simulink model "ACCSampleSimulink"  (R2022a)
settings: Solver=ode1  StartTime=0.0  StopTime=inf  FixedStep=0.001  RelTol=1e-3
model workspace (MAT data in the model file):
  ParaDataStoreNum : Simulink.Parameter (value not decoded)
undefined symbols (not defined in the file): azimuth_angle, DataStoreNumPara, elevation_angle, GroundTruth_Objects, heading, id, range_bbox, range_center, shape, time, type, velocity, width
(part 2 of 2)

== matlab function ACCSampleSimulink/Veh_1/ComplexVehicleModel/RoadInfo/MATLAB Function ==
  data: fl input; tire_x output; fr input; rl input; rr input; tire_y output; tire_z output
function [tire_x,tire_y,tire_z] = fcn(fl,fr,rl,rr)

tire_x = [fl(11),fr(11),rl(11),rr(11)];
tire_y = [fl(12),fr(12),rl(12),rr(12)];
tire_z = [fl(13),fr(13),rl(13),rr(13)];

== matlab function ACCSampleSimulink/Veh_1/ComplexVehicleModel/RoadInfo/MATLAB Function1 ==
  data: t input; outz output; z input; dzdx input; dzdy input; mu input; tirez input; outdzdx output; outdzdy output; outmu output
function [outz,outdzdx,outdzdy,outmu] = fcn(t,z,dzdx,dzdy,mu,tirez)
%#codegen
outz = tirez;
outdzdx = [0,0,0,0];
outdzdy = [0,0,0,0];
outmu = [0.75,0.75,0.75,0.75];
if t > 0.001
    outz = z;
    outdzdx = dzdx;
    outdzdy = dzdy;
    outmu = mu;
end

== matlab function ACCSampleSimulink/Veh_1/VehicleDataBus/MATLAB Function ==
  data: u input; head output; c_x output; c_y output; c_z output; yaw output; pitch output; roll output; rot_spd output; f_x output; f_y output; f_z output; g_x output; g_y output; g_z output
function [head,c_x,c_y,c_z,yaw,pitch,roll,rot_spd,f_x,f_y,f_z,g_x,g_y,g_z] = fcn(u)
head = [u(1),u(2),u(3),u(4),u(5)];
start = 6;
c_x =   [u(start),u(start+13),u(start+26),u(start+39)];
start = 7;
c_y =   [u(start),u(start+13),u(start+26),u(start+39)];
start = 8;
c_z =   [u(start),u(start+13),u(start+26),u(start+39)];
start = 9;
yaw =   [u(start),u(start+13),u(start+26),u(start+39)];
start = 10;
pitch = [u(start),u(start+13),u(start+26),u(start+39)];
start = 11;
roll =  [u(start),u(start+13),u(start+26),u(start+39)];
start = 12;
rot_spd =  [u(start),u(start+13),u(start+26),u(start+39)];
start = 13;
f_x =  [u(start),u(start+13),u(start+26),u(start+39)];
start = 14;
f_y =  [u(start),u(start+13),u(start+26),u(start+39)];
start = 15;
f_z =  [u(start),u(start+13),u(start+26),u(start+39)];
start = 16;
g_x =  [u(start),u(start+13),u(start+26),u(start+39)];
start = 17;
g_y =  [u(start),u(start+13),u(start+26),u(start+39)];
start = 18;
g_z =  [u(start),u(start+13),u(start+26),u(start+39)];

== matlab function ACCSampleSimulink/Veh_1/ComplexVehicleModel/MATLAB Function1 ==
  data: u input; ego output; egoextra output
function [ego,egoextra] = fcn(u)

ego = [u(2),u(3),u(4),u(5),u(6),u(7),u(8)];
egoextra = [u(8),u(9),u(10),u(11),u(12),u(13),u(14),u(15),u(16),u(17),u(18),u(19)];

== matlab function ACCSampleSimulink/Veh_1/ComplexVehicleModel/MATLAB Function2 ==
  data: driverControl input; throttle output; dynamicControl input; brake output; steer output; mode output
function [throttle,brake,steer,mode] = fcn(driverControl,dynamicControl)
%#codegen
if driverControl(1) > 0.5
    throttle = driverControl(2);
    brake = driverControl(3)* 1e6;
    steer = driverControl(4) * 0.0174;
    mode = driverControl(5);
else
    throttle = dynamicControl(3);
    brake = dynamicControl(4);
    steer = dynamicControl(5);
    mode = dynamicControl(2);
end

if mode > 0.5
   mode = 1 ;
end

== matlab function ACCSampleSimulink/Veh_1/Algorithm/ Find Leader Car/Find Leader Car ==
  data: EGOX input; RelatedDistance output; EGOY input; EGOV input; EGOYAW input; time input; width input; ids input; types input; shapes input; range_centers input; range_bboxs input; azimuth_angles input; elevation_angles input; velocitys input; headings input; RelatedSpeed output
function [RelatedDistance, RelatedSpeed]  = DetectionConcatenation(EGOX,EGOY,EGOV, EGOYAW, time, width, ids, types, shapes, range_centers, range_bboxs, azimuth_angles, elevation_angles, velocitys, headings)


% This function finds the lead car: a car in front of the ego car that
% satisfies all the criteria below:
% * Within the ego car's lane.
% * In front of the ego car.
% * Closest to the ego car.


% 1. The lane is defined using a parabolic model, where y=ax^2+bx+c. a is
%    equal to half the road curvature, b=0, and c is the offset of the lane
%    boundaries relative to the ego car. Overall lane width is assumed to
%    be 3.6m, typical highway lane width.
laneWidth = 3.6;

% 2. The ego car is assumed to be traveling in the middle of its lane, with
%    1.8m on each side of it. So, c=+1.8m for the left lane boundary and
%    -1.8m for the right lane boundary.
halfLaneWidth = laneWidth/2;

maxX = cast(500.0,'double');
Selected = cast(-1,'int32');

if(width > 0)
    for i = 1:width
        dis = range_bboxs(i);
        speed = velocitys(i);
        angle = -azimuth_angles(i);
        yaw = 3.1415926/2 - headings(i);
        deltaYaw = yaw - EGOYAW;
        x = dis * cos(angle); % Longitudinal position of the track relative to ego
        y = dis * sin(angle); % Lateral position of the track relative to ego
        if dis < maxX && dis > 0
            yleftLane  = polyval([0, 0,  halfLaneWidth],x); % Half a lane to the left
            yrightLane = polyval([0, 0, -halfLaneWidth],x); % Half a lane to the right

            % Find a new lead car
            if(yrightLane <= y) && (y<=yleftLane)
                maxX = cast(dis,'double');
                Selected = i;
            end
        end
    end
end

if(Selected ~= -1)
    RelatedDistance = cast(range_bboxs(Selected),'double');
    yaw = 3.1415926/2 - headings(Selected);
    speed = velocitys(Selected);
    deltaYaw = yaw - EGOYAW;
    Vxx = speed * cos(deltaYaw);
    %Vyy = speed * sin(deltaYaw);
    RelatedSpeed = cast(-EGOV + Vxx,'double');
else
    RelatedDistance = 500;
    RelatedSpeed = 0.1;
end

== matlab function ACCSampleSimulink/Veh_1/ComplexVehicleModel/RoadInfo/Subsystem/front_right ==
  data: out output double; xarry input; yarray input; zarray input; dzdxarray input; dzdyarray input; muarray input; x input; y input
function out  = fcn(xarry,yarray,zarray,dzdxarray,dzdyarray,muarray,x,y)
[x1,y1,x2,y2,x3,y3,x4,y4] = fcn_getpoint(xarry,yarray);
data_array = fcn_getdata(zarray,dzdxarray, dzdyarray,muarray);

zero = 0.001;
if ( abs(y2-y1) > zero )
   angle = 2*pi -  atan2(y2-y1,x2-x1);
   sin_angle = sin(angle);
   cos_angle = cos(angle);
   [x1,y1] = fcn_convert(x1,y1,x1,y1,sin_angle,cos_angle);
   [x2,y2] = fcn_convert(x1,y1,x2,y2,sin_angle,cos_angle);
   [x3,y3] = fcn_convert(x1,y1,x3,y3,sin_angle,cos_angle);
   [x4,y4] = fcn_convert(x1,y1,x4,y4,sin_angle,cos_angle);
   [x,y] = fcn_convert(x1,y1,x,y,sin_angle,cos_angle);
end

axle_x_left  = min(x1,x2);
axle_x_right = max(x1,x2);
axle_y_up    = max(y2,y3);
axle_y_down  = min(y2,y3);

% after rotota
% p1  p2
%
% p3 p4
z = 0;
dzdx = 0;
dzdy = 0;
mu = 0;
if ( x > axle_x_left ) && ( x < axle_x_right ) && ( y > axle_y_down ) && ( y < axle_y_up )
    xx1 = x3;
    xx2 = x4;
    yy1 = y3;
    yy2 = y1;
    matrix_left = [xx2-x  x-xx1];
    matrix_right = [ yy2 - y; y-yy1 ];
    delta = (xx2-xx1)*(yy2-yy1);
    delta = 1.0/delta;
    [z, dzdx, dzdy, mu] = fcn_cal(matrix_left,matrix_right,delta,data_array);
else
    if ( y >= axle_y_up ) 
        [z, dzdx, dzdy, mu] = fcn_cal_getmax(data_array(1,:),data_array(2,:));
    end
    if ( y <= axle_y_down )
        [z, dzdx, dzdy, mu] = fcn_cal_getmax(data_array(3,:),data_array(4,:));
    end
    if ( x >= axle_x_right )
        [z, dzdx, dzdy, mu] = fcn_cal_getmax(data_array(2,:),data_array(4,:));
    end
    if ( x <= axle_x_left )
        [z, dzdx, dzdy, mu] = fcn_cal_getmax(data_array(1,:),data_array(3,:));
    end
end

out = [z dzdx dzdy mu];
end

function [xxx,yyy] = fcn_convert(x0,y0,x1,y1,sin_agnle,cos_angle)
    xxx = (x1-x0)*cos_angle - (y1-y0)*sin_agnle + x0;
    yyy = (x1-x0)*sin_agnle + (y1-y0)*cos_angle + y0;
end

function [x1,y1,x2,y2,x3,y3,x4,y4] = fcn_getpoint(xarry,yarray)
    x1 = xarry(1);
    x2 = xarry(2);
    x3 = xarry(3);
    x4 = xarry(4);
    y1 = yarray(1);
    y2 = yarray(2);
    y3 = yarray(3);
    y4 = yarray(4);
end

function ret = fcn_getdata(zarray,dzdxarray, dzdyarray,muarray)
    ret = [ 
        zarray(1),dzdxarray(1),dzdyarray(1),muarray(1);
        zarray(2),dzdxarray(2),dzdyarray(2),muarray(2);
        zarray(3),dzdxarray(3),dzdyarray(3),muarray(3);
        zarray(4),dzdxarray(4),dzdyarray(4),muarray(4);
    ];
end

function [z,dzdx,dzdy,mu] = fcn_cal(matrix_left,matrix_right , delta, data_array)
%matrix_z = [z3, z1; z4 , z2]
%value = [xx2-x  x-xx1] * matrix * [ yy2 - y; y-yy1 ]  * d1
    array_z = data_array(:,1);
    array_dzdx = data_array(:,2);
    array_dzdy = data_array(:,3);
    array_mu = data_array(:,4);
    z = matrix_left * [array_z(3), array_z(1); array_z(4),array_z(2)] * matrix_right  * delta;
    dzdx = matrix_left * [array_dzdx(3), array_dzdx(1); array_dzdx(4),array_dzdx(2)] * matrix_right  * delta;
    dzdy = matrix_left * [array_dzdy(3), array_dzdy(1); array_dzdy(4),array_dzdy(2)] * matrix_right  * delta;
    mu = matrix_left * [array_mu(3), array_mu(1); array_mu(4),array_mu(2)] * matrix_right  * delta;
end

function [z,dzdx,dzdy,mu] = fcn_cal_getmax(data1,data2)
    z = max(data1(1),data2(1));
    dzdx = max(data1(2),data2(2));
    dzdy = max(data1(3),data2(3));
    mu = max(data1(4),data2(4));
end

== matlab function ACCSampleSimulink/Veh_1/ComplexVehicleModel/RoadInfo/Subsystem/front_left ==
  data: out output double; xarry input; yarray input; zarray input; dzdxarray input; dzdyarray input; muarray input; x input; y input
function out  = fcn(xarry,yarray,zarray,dzdxarray,dzdyarray,muarray,x,y)
[x1,y1,x2,y2,x3,y3,x4,y4] = fcn_getpoint(xarry,yarray);
data_array = fcn_getdata(zarray,dzdxarray, dzdyarray,muarray);

zero = 0.001;
if ( abs(y2-y1) > zero )
   angle = 2*pi -  atan2(y2-y1,x2-x1);
   sin_angle = sin(angle);
   cos_angle = cos(angle);
   [x1,y1] = fcn_convert(x1,y1,x1,y1,sin_angle,cos_angle);
   [x2,y2] = fcn_convert(x1,y1,x2,y2,sin_angle,cos_angle);
   [x3,y3] = fcn_convert(x1,y1,x3,y3,sin_angle,cos_angle);
   [x4,y4] = fcn_convert(x1,y1,x4,y4,sin_angle,cos_angle);
   [x,y] = fcn_convert(x1,y1,x,y,sin_angle,cos_angle);
end

axle_x_left  = min(x1,x2);
axle_x_right = max(x1,x2);
axle_y_up    = max(y2,y3);
axle_y_down  = min(y2,y3);

% after rotota
% p1  p2
%
% p3 p4
z = 0;
dzdx = 0;
dzdy = 0;
mu = 0;
if ( x > axle_x_left ) && ( x < axle_x_right ) && ( y > axle_y_down ) && ( y < axle_y_up )
    xx1 = x3;
    xx2 = x4;
    yy1 = y3;
    yy2 = y1;
    matrix_left = [xx2-x  x-xx1];
    matrix_right = [ yy2 - y; y-yy1 ];
    delta = (xx2-xx1)*(yy2-yy1);
    delta = 1.0/delta;
    [z, dzdx, dzdy, mu] = fcn_cal(matrix_left,matrix_right,delta,data_array);
else
    if ( y >= axle_y_up ) 
        [z, dzdx, dzdy, mu] = fcn_cal_getmax(data_array(1,:),data_array(2,:));
    end
    if ( y <= axle_y_down )
        [z, dzdx, dzdy, mu] = fcn_cal_getmax(data_array(3,:),data_array(4,:));
    end
    if ( x >= axle_x_right )
        [z, dzdx, dzdy, mu] = fcn_cal_getmax(data_array(2,:),data_array(4,:));
    end
    if ( x <= axle_x_left )
        [z, dzdx, dzdy, mu] = fcn_cal_getmax(data_array(1,:),data_array(3,:));
    end
end

out = [z dzdx dzdy mu];
end

function [xxx,yyy] = fcn_convert(x0,y0,x1,y1,sin_agnle,cos_angle)
    xxx = (x1-x0)*cos_angle - (y1-y0)*sin_agnle + x0;
    yyy = (x1-x0)*sin_agnle + (y1-y0)*cos_angle + y0;
end

function [x1,y1,x2,y2,x3,y3,x4,y4] = fcn_getpoint(xarry,yarray)
    x1 = xarry(1);
    x2 = xarry(2);
    x3 = xarry(3);
    x4 = xarry(4);
    y1 = yarray(1);
    y2 = yarray(2);
    y3 = yarray(3);
    y4 = yarray(4);
end

function ret = fcn_getdata(zarray,dzdxarray, dzdyarray,muarray)
    ret = [ 
        zarray(1),dzdxarray(1),dzdyarray(1),muarray(1);
        zarray(2),dzdxarray(2),dzdyarray(2),muarray(2);
        zarray(3),dzdxarray(3),dzdyarray(3),muarray(3);
        zarray(4),dzdxarray(4),dzdyarray(4),muarray(4);
    ];
end

function [z,dzdx,dzdy,mu] = fcn_cal(matrix_left,matrix_right , delta, data_array)
%matrix_z = [z3, z1; z4 , z2]
%value = [xx2-x  x-xx1] * matrix * [ yy2 - y; y-yy1 ]  * d1
    array_z = data_array(:,1);
    array_dzdx = data_array(:,2);
    array_dzdy = data_array(:,3);
    array_mu = data_array(:,4);
    z = matrix_left * [array_z(3), array_z(1); array_z(4),array_z(2)] * matrix_right  * delta;
    dzdx = matrix_left * [array_dzdx(3), array_dzdx(1); array_dzdx(4),array_dzdx(2)] * matrix_right  * delta;
    dzdy = matrix_left * [array_dzdy(3), array_dzdy(1); array_dzdy(4),array_dzdy(2)] * matrix_right  * delta;
    mu = matrix_left * [array_mu(3), array_mu(1); array_mu(4),array_mu(2)] * matrix_right  * delta;
end

function [z,dzdx,dzdy,mu] = fcn_cal_getmax(data1,data2)
    z = max(data1(1),data2(1));
    dzdx = max(data1(2),data2(2));
    dzdy = max(data1(3),data2(3));
    mu = max(data1(4),data2(4));
end

== matlab function ACCSampleSimulink/Veh_1/ComplexVehicleModel/RoadInfo/Subsystem/tail_left ==
  data: out output double; xarry input; yarray input; zarray input; dzdxarray input; dzdyarray input; muarray input; x input; y input
function out  = fcn(xarry,yarray,zarray,dzdxarray,dzdyarray,muarray,x,y)
[x1,y1,x2,y2,x3,y3,x4,y4] = fcn_getpoint(xarry,yarray);
data_array = fcn_getdata(zarray,dzdxarray, dzdyarray,muarray);

zero = 0.001;
if ( abs(y2-y1) > zero )
   angle = 2*pi -  atan2(y2-y1,x2-x1);
   sin_angle = sin(angle);
   cos_angle = cos(angle);
   [x1,y1] = fcn_convert(x1,y1,x1,y1,sin_angle,cos_angle);
   [x2,y2] = fcn_convert(x1,y1,x2,y2,sin_angle,cos_angle);
   [x3,y3] = fcn_convert(x1,y1,x3,y3,sin_angle,cos_angle);
   [x4,y4] = fcn_convert(x1,y1,x4,y4,sin_angle,cos_angle);
   [x,y] = fcn_convert(x1,y1,x,y,sin_angle,cos_angle);
end

axle_x_left  = min(x1,x2);
axle_x_right = max(x1,x2);
axle_y_up    = max(y2,y3);
axle_y_down  = min(y2,y3);

% after rotota
% p1  p2
%
% p3 p4
z = 0;
dzdx = 0;
dzdy = 0;
mu = 0;
if ( x > axle_x_left ) && ( x < axle_x_right ) && ( y > axle_y_down ) && ( y < axle_y_up )
    xx1 = x3;
    xx2 = x4;
    yy1 = y3;
    yy2 = y1;
    matrix_left = [xx2-x  x-xx1];
    matrix_right = [ yy2 - y; y-yy1 ];
    delta = (xx2-xx1)*(yy2-yy1);
    delta = 1.0/delta;
    [z, dzdx, dzdy, mu] = fcn_cal(matrix_left,matrix_right,delta,data_array);
else
    if ( y >= axle_y_up ) 
        [z, dzdx, dzdy, mu] = fcn_cal_getmax(data_array(1,:),data_array(2,:));
    end
    if ( y <= axle_y_down )
        [z, dzdx, dzdy, mu] = fcn_cal_getmax(data_array(3,:),data_array(4,:));
    end
    if ( x >= axle_x_right )
        [z, dzdx, dzdy, mu] = fcn_cal_getmax(data_array(2,:),data_array(4,:));
    end
    if ( x <= axle_x_left )
        [z, dzdx, dzdy, mu] = fcn_cal_getmax(data_array(1,:),data_array(3,:));
    end
end

out = [z dzdx dzdy mu];
end

function [xxx,yyy] = fcn_convert(x0,y0,x1,y1,sin_agnle,cos_angle)
    xxx = (x1-x0)*cos_angle - (y1-y0)*sin_agnle + x0;
    yyy = (x1-x0)*sin_agnle + (y1-y0)*cos_angle + y0;
end

function [x1,y1,x2,y2,x3,y3,x4,y4] = fcn_getpoint(xarry,yarray)
    x1 = xarry(1);
    x2 = xarry(2);
    x3 = xarry(3);
    x4 = xarry(4);
    y1 = yarray(1);
    y2 = yarray(2);
    y3 = yarray(3);
    y4 = yarray(4);
end

function ret = fcn_getdata(zarray,dzdxarray, dzdyarray,muarray)
    ret = [ 
        zarray(1),dzdxarray(1),dzdyarray(1),muarray(1);
        zarray(2),dzdxarray(2),dzdyarray(2),muarray(2);
        zarray(3),dzdxarray(3),dzdyarray(3),muarray(3);
        zarray(4),dzdxarray(4),dzdyarray(4),muarray(4);
    ];
end

function [z,dzdx,dzdy,mu] = fcn_cal(matrix_left,matrix_right , delta, data_array)
%matrix_z = [z3, z1; z4 , z2]
%value = [xx2-x  x-xx1] * matrix * [ yy2 - y; y-yy1 ]  * d1
    array_z = data_array(:,1);
    array_dzdx = data_array(:,2);
    array_dzdy = data_array(:,3);
    array_mu = data_array(:,4);
    z = matrix_left * [array_z(3), array_z(1); array_z(4),array_z(2)] * matrix_right  * delta;
    dzdx = matrix_left * [array_dzdx(3), array_dzdx(1); array_dzdx(4),array_dzdx(2)] * matrix_right  * delta;
    dzdy = matrix_left * [array_dzdy(3), array_dzdy(1); array_dzdy(4),array_dzdy(2)] * matrix_right  * delta;
    mu = matrix_left * [array_mu(3), array_mu(1); array_mu(4),array_mu(2)] * matrix_right  * delta;
end

function [z,dzdx,dzdy,mu] = fcn_cal_getmax(data1,data2)
    z = max(data1(1),data2(1));
    dzdx = max(data1(2),data2(2));
    dzdy = max(data1(3),data2(3));
    mu = max(data1(4),data2(4));
end

== matlab function ACCSampleSimulink/Veh_1/ComplexVehicleModel/RoadInfo/Subsystem/tail_right ==
  data: out output double; xarry input; yarray input; zarray input; dzdxarray input; dzdyarray input; muarray input; x input; y input
function out  = fcn(xarry,yarray,zarray,dzdxarray,dzdyarray,muarray,x,y)
[x1,y1,x2,y2,x3,y3,x4,y4] = fcn_getpoint(xarry,yarray);
data_array = fcn_getdata(zarray,dzdxarray, dzdyarray,muarray);

zero = 0.001;
if ( abs(y2-y1) > zero )
   angle = 2*pi -  atan2(y2-y1,x2-x1);
   sin_angle = sin(angle);
   cos_angle = cos(angle);
   [x1,y1] = fcn_convert(x1,y1,x1,y1,sin_angle,cos_angle);
   [x2,y2] = fcn_convert(x1,y1,x2,y2,sin_angle,cos_angle);
   [x3,y3] = fcn_convert(x1,y1,x3,y3,sin_angle,cos_angle);
   [x4,y4] = fcn_convert(x1,y1,x4,y4,sin_angle,cos_angle);
   [x,y] = fcn_convert(x1,y1,x,y,sin_angle,cos_angle);
end

axle_x_left  = min(x1,x2);
axle_x_right = max(x1,x2);
axle_y_up    = max(y2,y3);
axle_y_down  = min(y2,y3);

% after rotota
% p1  p2
%
% p3 p4
z = 0;
dzdx = 0;
dzdy = 0;
mu = 0;
if ( x > axle_x_left ) && ( x < axle_x_right ) && ( y > axle_y_down ) && ( y < axle_y_up )
    xx1 = x3;
    xx2 = x4;
    yy1 = y3;
    yy2 = y1;
    matrix_left = [xx2-x  x-xx1];
    matrix_right = [ yy2 - y; y-yy1 ];
    delta = (xx2-xx1)*(yy2-yy1);
    delta = 1.0/delta;
    [z, dzdx, dzdy, mu] = fcn_cal(matrix_left,matrix_right,delta,data_array);
else
    if ( y >= axle_y_up ) 
        [z, dzdx, dzdy, mu] = fcn_cal_getmax(data_array(1,:),data_array(2,:));
    end
    if ( y <= axle_y_down )
        [z, dzdx, dzdy, mu] = fcn_cal_getmax(data_array(3,:),data_array(4,:));
    end
    if ( x >= axle_x_right )
        [z, dzdx, dzdy, mu] = fcn_cal_getmax(data_array(2,:),data_array(4,:));
    end
    if ( x <= axle_x_left )
        [z, dzdx, dzdy, mu] = fcn_cal_getmax(data_array(1,:),data_array(3,:));
    end
end

out = [z dzdx dzdy mu];
end

function [xxx,yyy] = fcn_convert(x0,y0,x1,y1,sin_agnle,cos_angle)
    xxx = (x1-x0)*cos_angle - (y1-y0)*sin_agnle + x0;
    yyy = (x1-x0)*sin_agnle + (y1-y0)*cos_angle + y0;
end

function [x1,y1,x2,y2,x3,y3,x4,y4] = fcn_getpoint(xarry,yarray)
    x1 = xarry(1);
    x2 = xarry(2);
    x3 = xarry(3);
    x4 = xarry(4);
    y1 = yarray(1);
    y2 = yarray(2);
    y3 = yarray(3);
    y4 = yarray(4);
end

function ret = fcn_getdata(zarray,dzdxarray, dzdyarray,muarray)
    ret = [ 
        zarray(1),dzdxarray(1),dzdyarray(1),muarray(1);
        zarray(2),dzdxarray(2),dzdyarray(2),muarray(2);
        zarray(3),dzdxarray(3),dzdyarray(3),muarray(3);
        zarray(4),dzdxarray(4),dzdyarray(4),muarray(4);
    ];
end

function [z,dzdx,dzdy,mu] = fcn_cal(matrix_left,matrix_right , delta, data_array)
%matrix_z = [z3, z1; z4 , z2]
%value = [xx2-x  x-xx1] * matrix * [ yy2 - y; y-yy1 ]  * d1
    array_z = data_array(:,1);
    array_dzdx = data_array(:,2);
    array_dzdy = data_array(:,3);
    array_mu = data_array(:,4);
    z = matrix_left * [array_z(3), array_z(1); array_z(4),array_z(2)] * matrix_right  * delta;
    dzdx = matrix_left * [array_dzdx(3), array_dzdx(1); array_dzdx(4),array_dzdx(2)] * matrix_right  * delta;
    dzdy = matrix_left * [array_dzdy(3), array_dzdy(1); array_dzdy(4),array_dzdy(2)] * matrix_right  * delta;
    mu = matrix_left * [array_mu(3), array_mu(1); array_mu(4),array_mu(2)] * matrix_right  * delta;
end

function [z,dzdx,dzdy,mu] = fcn_cal_getmax(data1,data2)
    z = max(data1(1),data2(1));
    dzdx = max(data1(2),data2(2));
    dzdy = max(data1(3),data2(3));
    mu = max(data1(4),data2(4));
end
